simulink model "AdaptiveSigmaDelta"  (R2020a)
settings: Solver=VariableStepAuto  StartTime=0.0  StopTime=10.0  RelTol=1e-3
undefined symbols (not defined in the file): DiscIntNeverNeededParam
settings Model: Creator=diflo  LastModifiedBy=diflo

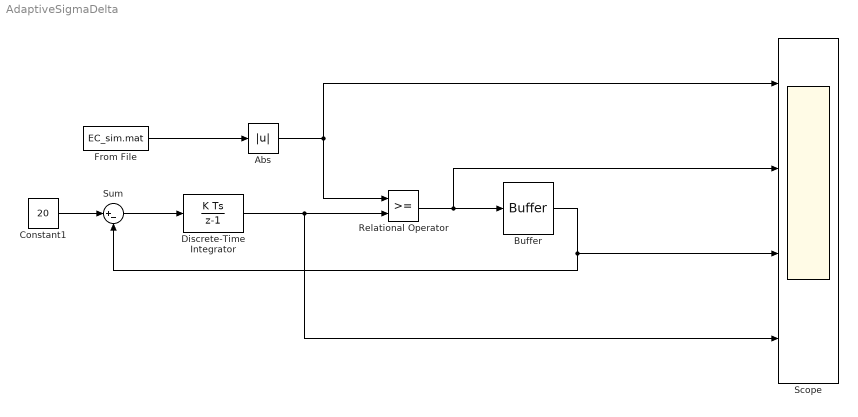
== system AdaptiveSigmaDelta ==
  Abs : Abs
  Buffer : Buffer  N=128  OutputFrames=off
  Constant1 : Constant  Value=20  SampleTime=1/30000
  Discrete-Time Integrator : DiscreteIntegrator  SampleTime=1/30000  ICPrevOutput=DiscIntNeverNeededParam  ICPrevScaledInput=DiscIntNeverNeededParam
  From File : FromFile  FileName=EC_sim.mat  SampleTime=1/30000
  Relational Operator : RelationalOperator  OutDataTypeStr=boolean
  Scope : Scope  NumInputPorts=4
  Sum : Sum  Inputs=|+-
  wires:
  From File/1 -> Abs/1
  Abs/1 -> Scope/1, Relational Operator/1
  Discrete-Time Integrator/1 -> Scope/4, Relational Operator/2
  Sum/1 -> Discrete-Time Integrator/1
  Constant1/1 -> Sum/1
  Relational Operator/1 -> Scope/2, Buffer/1
  Buffer/1 -> Scope/3, Sum/2
